simulink model "system"  (R2013b)
settings: Solver=ode45  StartTime=0  StopTime=2  RelTol=1e-3
settings Model: Creator=erich  LastModifiedBy=erich

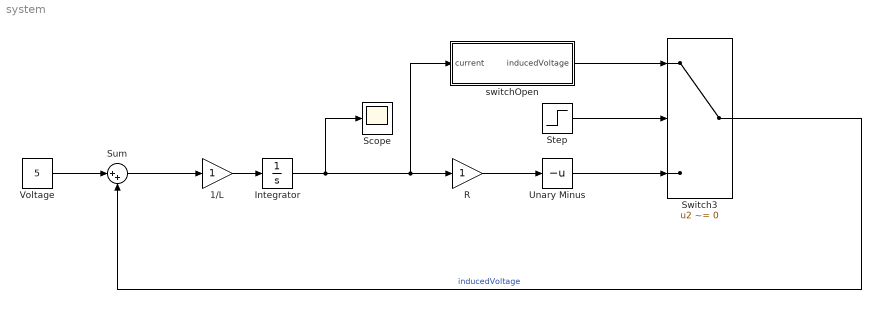
== system system ==
  1/L : Gain
  Integrator : Integrator
      settings: AttributesFormatString=x0: %<InitialCondition>
  R : Gain
  Scope : Scope
  Step : Step  SampleTime=0
  Sum : Sum  Inputs=|++
  Switch3 : Switch  Criteria=u2 ~= 0
  Unary Minus : UnaryMinus
  Voltage : Constant  Value=5
  switchOpen : Subsystem
  wires:
  Voltage/1 -> Sum/1
  Sum/1 -> 1/L/1
  1/L/1 -> Integrator/1
  Switch3/1 -> Sum/2  "inducedVoltage"
  Step/1 -> Switch3/2
  switchOpen/1(inducedVoltage) -> Switch3/1
  R/1 -> Unary Minus/1
  Unary Minus/1 -> Switch3/3
  Integrator/1 -> Scope/1, switchOpen/1(current), R/1

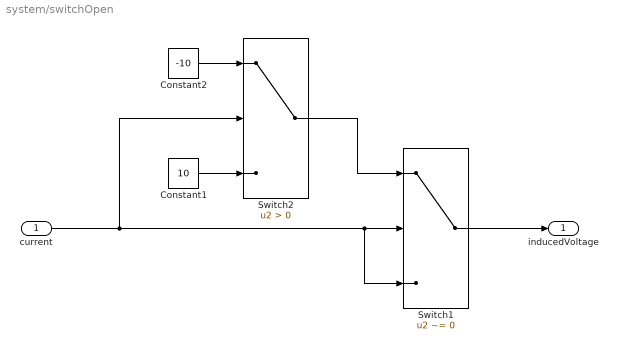
== system system/switchOpen ==
  current : Inport
  Constant1 : Constant  Value=10
  Constant2 : Constant  Value=-10
  Switch1 : Switch  Criteria=u2 ~= 0
  Switch2 : Switch  Criteria=u2 > Threshold
  inducedVoltage : Outport
  wires:
  Switch1/1 -> inducedVoltage/1
  current/1 -> Switch1/3, Switch1/2, Switch2/2
  Constant2/1 -> Switch2/1
  Switch2/1 -> Switch1/1
  Constant1/1 -> Switch2/3
